simulink model "eskf_block"  (R2025b)
settings: Solver=FixedStepDiscrete  StartTime=0.0  StopTime=5  FixedStep=0.0024  RelTol=1e-3
settings Model: Creator=Ashwin  LastModifiedBy=Ashwin

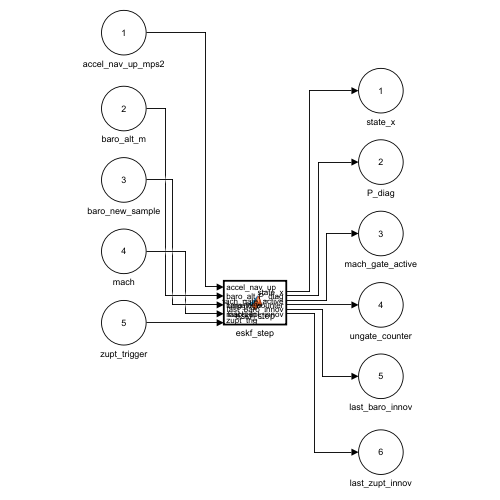
[thumbnail: Simulink's stored preview of the top-level diagram]
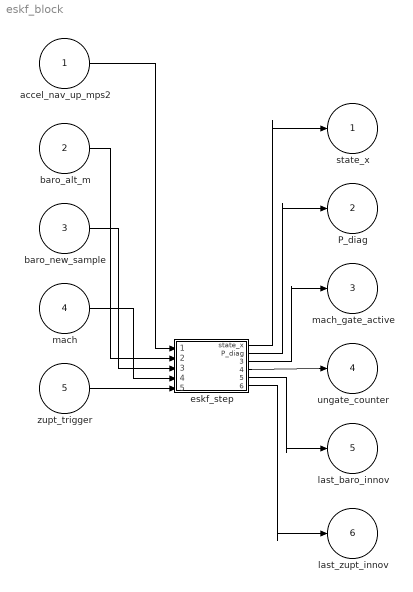
== system eskf_block ==
  accel_nav_up_mps2 : Inport  SampleTime=0.0024
  baro_alt_m : Inport  Port=2  SampleTime=0.01
  baro_new_sample : Inport  Port=3  SampleTime=0.01
  mach : Inport  Port=4  SampleTime=0.0024
  zupt_trigger : Inport  Port=5  SampleTime=0.0024
  eskf_step : MATLAB Function  TreatAsAtomicUnit=on
  state_x : Outport
  P_diag : Outport  Port=2
  mach_gate_active : Outport  Port=3
  ungate_counter : Outport  Port=4
  last_baro_innov : Outport  Port=5
  last_zupt_innov : Outport  Port=6
  wires:
  accel_nav_up_mps2/1 -> eskf_step/1(accel_nav_up)
  baro_alt_m/1 -> eskf_step/2(baro_alt)
  baro_new_sample/1 -> eskf_step/3(baro_new)
  mach/1 -> eskf_step/4(mach_in)
  zupt_trigger/1 -> eskf_step/5(zupt_trig)
  eskf_step/1(state_x) -> state_x/1
  eskf_step/3(mach_gate_active) -> mach_gate_active/1
  eskf_step/2(P_diag) -> P_diag/1
  eskf_step/4(ungate_counter) -> ungate_counter/1
  eskf_step/5(last_baro_innov) -> last_baro_innov/1
  eskf_step/6(last_zupt_innov) -> last_zupt_innov/1

== matlab function eskf_block/eskf_step ==
  data: accel_nav_up input; state_x output; baro_alt input; baro_new input; mach_in input; zupt_trig input; P_diag output; mach_gate_active output; ungate_counter output; last_baro_innov output; last_zupt_innov output
function [state_x, P_diag, mach_gate_active, ungate_counter, last_baro_innov, last_zupt_innov] = eskf_step(accel_nav_up, baro_alt, baro_new, mach_in, zupt_trig)
% Persistent ESKF state container. Reset via subsystem Init callback.
persistent st Est
if isempty(st)
    casper_sensor_params; %#ok<NASGU>
    Est = evalin('base', 'Estimator');
    st = casper_eskf_state('init', Est, baro_alt);
end
% Predict (every call)
st = casper_eskf_predict(st, accel_nav_up, Est);
% Mach gate (every call)
st = casper_eskf_mach_gate(st, mach_in, Est);
% Baro update (when new baro sample)
if baro_new
    st = casper_eskf_update_baro(st, baro_alt, Est);
end
% ZUPT update
if zupt_trig
    st = casper_eskf_update_zupt(st, Est);
end
state_x = st.x_vec;
P_diag = diag(st.P_mat);
mach_gate_active = double(st.mach_gate_active);
ungate_counter = double(st.ungate_counter);
last_baro_innov = st.last_baro_innov_m;
last_zupt_innov = st.last_zupt_innov_mps;
end
